simulink model "proje4__SIP_DynSys_Model_V2_0"  (R2024a)
settings: Solver=FixedStepAuto  StartTime=0.0  StopTime=10  FixedStep=0.001  RelTol=1e-3
undefined symbols (not defined in the file): motorForces, motorTorques, q_dot_InitCond, q_InitCond, systemConstant, X, Y, Z
libraries: sm_lib x41, nesl_utility x13
(part 2 of 2)

== matlab function proje4__SIP_DynSys_Model_V2_0/DroneDynamics ==
  data: q input; q_ddot output; q_dot input; systemConstant input; motorForces input; motorTorques input
    function q_ddot = fcn(q, q_dot, systemConstant, motorForces, motorTorques)
  q_ddot = zeros(8, 1); % Boyut sabit: 8x1

%% ====[ System Constants ]====

M_drone = systemConstant(1);   % kg, Mass of the drone (without pendulum)
mc      = systemConstant(2);   % kg, Mass of the pendulum (without drone)
l       = systemConstant(3);   % m,  Length of the pendulum stick
g       = 9.81;                % m/s^2, Gravitational acceleration
DroneArmLength = systemConstant(4); %m, Distance from the center of the drone to the center of the motor 

% Thrust force per motor
MotorForce_1 = motorForces(1); 
MotorForce_2 = motorForces(2);
MotorForce_3 = motorForces(3);
MotorForce_4 = motorForces(4);
force_total      = MotorForce_1 + MotorForce_2 + MotorForce_3 + MotorForce_4; 

% Thrust Torque per motor
MotorTorque_1 = motorTorques(1);
MotorTorque_2 = motorTorques(2);
MotorTorque_3 = motorTorques(3);
MotorTorque_4 = motorTorques(4);
%torque_total = MotorTorque_1 + MotorTorque_2 + MotorTorque_3 + MotorTorque_4;
    %Changed sign of the variable MotorTorque 2 and 4, because of its
    %rotations are CW, other ones are CCW, they are opposite of each other 
torque_total = MotorTorque_1 - MotorTorque_2 + MotorTorque_3 - MotorTorque_4;

% Roll, pitch, and yaw torques applied to the frame
Torque_phi   = (MotorForce_2-MotorForce_4)*DroneArmLength;
Torque_theta = (MotorForce_3-MotorForce_1)*DroneArmLength;
Torque_psi  = (torque_total);


%% ====[ State Variable Extraction ]====
% Extract values and their derivatives from q and q_dot arrays 
% and assign them to respective physical quantities

% Content of q array ==> [x; y; z; fi; teta; psi; alfa; beta]
%                    ==> [q(1); q(2); q(3); q(4); q(5); q(6); q(7); q(8)]
% derivatives        ==> [x_dot; y_dot; z_dot; phi_dot; theta_dot; psi_dot; alfa_dot; beta_dot]
%                    ==> [q_dot(1); q_dot(2); q_dot(3); q_dot(4); q_dot(5); q_dot(6); q_dot(7); q_dot(8)]

x     = q(1);     x_dot = q_dot(1);     % x position and its derivative
y     = q(2);     y_dot = q_dot(2);     % y position and its derivative
z     = q(3);     z_dot = q_dot(3);     % z position and its derivative
phi   = q(4);   phi_dot = q_dot(4);     % phi angle and its derivative
theta = q(5); theta_dot = q_dot(5);     % theta angle and its derivative
psi   = q(6);   psi_dot = q_dot(6);     % psi angle and its derivative
alfa  = q(7);  alfa_dot = q_dot(7);     % alfa angle and its derivative
beta  = q(8);  beta_dot = q_dot(8);     % beta angle and its derivative


%% ====[ Trigonometric Shorthand Notations ]====
% To simplify the mathematical model representation, the following notation is used

C_alpha = cos(alfa);
S_alpha = sin(alfa);
C_beta  = cos(beta);
S_beta  = sin(beta);

C_phi   = cos(phi);
S_phi   = sin(phi);
C_theta = cos(theta);
S_theta = sin(theta);
C_psi   = cos(psi);
S_psi   = sin(psi);

%% ====[ SUBMATRICES FOR SYSTEM MATRIX M,C,G and B ]====  

% ------------------------------------------------------------------------%
%               Submatrices Contained in the System Matrix B              %
% ------------------------------------------------------------------------%

    % Matrix e
    M_e   = [0;
             0;
             1];

 
    % ZYX Euler açılarından rotasyon matrisi (body → inertial)==>ÇALIŞIYOR
    M_R = [...
        C_psi*C_theta,    C_psi*S_theta*S_phi - S_psi*C_phi,   C_psi*S_theta*C_phi + S_psi*S_phi;
        S_psi*C_theta,    S_psi*S_theta*S_phi + C_psi*C_phi,   S_psi*S_theta*C_phi - C_psi*S_phi;
        -S_theta     ,    C_theta*S_phi                    ,   C_theta*C_phi ];





% ------------------------------------------------------------------------%
%               Submatrices Contained in the System Matrix G              %
% ------------------------------------------------------------------------%
    
    % Matrix gmu
    M_gmu   = [-mc*l*g*S_alpha;
                      0      ];


% ------------------------------------------------------------------------%
%               Submatrices Contained in the System Matrix C              %
% ------------------------------------------------------------------------%
    
    % Matrix Psi
    M_Psi   = (mc*(l^2))*[         0             , -beta_dot*S_alpha*C_alpha;
                          beta_dot*S_alpha*C_beta, alfa_dot*S_alpha*C_beta ];
    
    % Matrix Gamma
    M_Gamma = (mc*l)*[-(alfa_dot*S_alpha + beta_dot*C_alpha*S_beta), -(alfa_dot*C_alpha*C_beta + beta_dot*S_alpha);
                      -(alfa_dot*S_alpha + beta_dot*C_alpha*S_beta), -(alfa_dot*C_alpha*C_beta + beta_dot*S_alpha);
                            -alfa_dot*C_alpha               ,                       0                            ];


% ------------------------------------------------------------------------%
%               Submatrices Contained in the System Matrix M              %
% ------------------------------------------------------------------------%
    
    % Matrix Theta
    M_theta = (mc*l)*[C_alpha*C_beta, -S_alpha*S_beta;
                      C_alpha*S_beta,  S_alpha*C_beta;
                      S_alpha       ,        0       ];

    % Matrix Tau(Transposed version)
    M_Tau   = (mc*l)*[C_alpha*C_beta , -C_alpha*S_beta, -S_alpha;
                      -S_alpha*S_beta,  S_alpha*C_beta,     0  ];

    % Matrix Phi
    M_Phi   = [mc*l^2,          0           ;
                 0   , mc*(l^2)*(S_alpha^2)];


%% ====[ SYSTEM MATRIX M,C,G,U and B ]====  
% q_ddot = M \ (B*U - C*q_dot - G );

% ------------------------------------------------------------------------%
%                                Matrix B                                 %
% ------------------------------------------------------------------------%
    
    B =  [M_R*M_e  , zeros(3,3) ;
         zeros(3,1),   eye(3)   ;
         zeros(2,1), zeros(2,3)];

% ------------------------------------------------------------------------%
%                                Matrix G                                 %
% ------------------------------------------------------------------------%
    
    G = [   zeros(2,1)  ;
        g*(M_drone + mc);
            zeros(3,1)  ;
              M_gmu    ];

% ------------------------------------------------------------------------%
%                                Matrix C                                 %
% ------------------------------------------------------------------------%
    
    C = [zeros(3,3), zeros(3,3), M_Gamma   ;
         zeros(3,3), zeros(3,3), zeros(3,2);
         zeros(2,3), zeros(2,3), M_Psi    ];

% ------------------------------------------------------------------------%
%                                Matrix M                                 %
% ------------------------------------------------------------------------%

    M = [(M_drone+mc)*eye(3), zeros(3,3) , M_theta   ;
            zeros(3,3)      ,   eye(3)   , zeros(3,2);
              M_Tau         , zeros(2,3) ,  M_Phi   ];

% ------------------------------------------------------------------------%
%                                Matrix U                                 %
% ------------------------------------------------------------------------%
U =[force_total;Torque_phi;Torque_theta;Torque_psi];




%% ====[ SOLVING SYSTEM DYNAMIC EQUATION ]====  
% 
 %q_ddot(:) = M \ (B*U - C*q_dot - G ); 
 q_ddot = pinv(M) * (B*U - C*q_dot - G);  


end
